simulink library "My_library"  (R2018a)
settings: Solver=VariableStepAuto  StartTime=0.0  StopTime=10.0  RelTol=1e-3  EnableMultiTasking=on
undefined symbols (not defined in the file or in its folder): Ax, Ay, Az, gn, Newton, Nx, Ny, Nz, Raphson, Rx, Ry, Rz, st
libraries: $bdroot x11, simulink x1
(part 2 of 2)

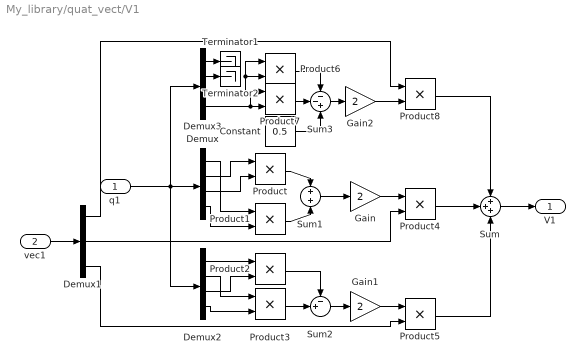
== system My_library/quat_vect/V1 ==
  q1 : Inport
  vec1 : Inport  Port=2
  Constant : Constant  Value=0.5
  Demux : Demux
  Demux1 : Demux  Outputs=3
  Demux2 : Demux
  Demux3 : Demux
  Gain : Gain  Gain=2
  Gain1 : Gain  Gain=2
  Gain2 : Gain  Gain=2
  Product{,1..8} (9 alike) : Product  RndMeth=Zero
  Sum : Sum  Inputs=3
  Sum1 : Sum  Inputs=+|+
  Sum2 : Sum  Inputs=-+|
  Sum3 : Sum  Inputs=--+
  Terminator1 : Terminator
  Terminator2 : Terminator
  V1 : Outport
  wires:
  q1/1 -> Demux2/1, Demux3/1, Demux/1
  Gain1/1 -> Product5/1
  Demux3/4 -> Product7/1, Product7/2
  Product4/1 -> Sum/2
  Product6/1 -> Sum3/1
  Demux/4 -> Product1/2
  Gain2/1 -> Product8/2
  Demux/3 -> Product/2
  Demux1/3 -> Product5/2
  Product8/1 -> Sum/1
  Demux1/2 -> Product4/2
  Demux/2 -> Product/1
  Demux1/1 -> Product8/1
  Sum1/1 -> Gain/1
  Demux2/3 -> Product2/2
  Demux3/3 -> Product6/2, Product6/1
  Constant/1 -> Sum3/3
  Demux3/2 -> Terminator2/1
  Demux3/1 -> Terminator1/1
  Sum3/1 -> Gain2/1
  Product1/1 -> Sum1/2
  Gain/1 -> Product4/1
  Demux2/4 -> Product3/2
  Demux2/1 -> Product2/1
  Product3/1 -> Sum2/2
  Product7/1 -> Sum3/2
  Demux2/2 -> Product3/1
  Product5/1 -> Sum/3
  Product/1 -> Sum1/1
  Demux/1 -> Product1/1
  Sum2/1 -> Gain1/1
  Sum/1 -> V1/1
  Product2/1 -> Sum2/1
  vec1/1 -> Demux1/1

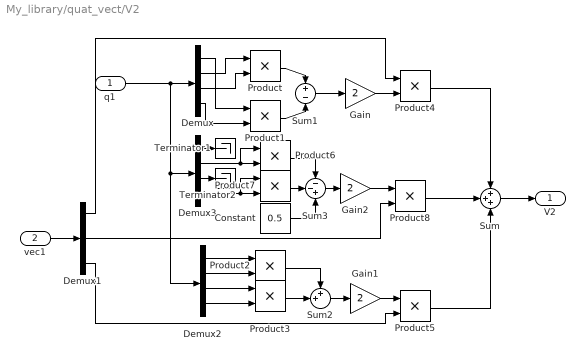
== system My_library/quat_vect/V2 ==
  q1 : Inport
  vec1 : Inport  Port=2
  Constant : Constant  Value=0.5
  Demux : Demux
  Demux1 : Demux  Outputs=3
  Demux2 : Demux
  Demux3 : Demux
  Gain : Gain  Gain=2
  Gain1 : Gain  Gain=2
  Gain2 : Gain  Gain=2
  Product{,1..8} (9 alike) : Product  RndMeth=Zero
  Sum : Sum  Inputs=3
  Sum1 : Sum  Inputs=+|-
  Sum2 : Sum  Inputs=++|
  Sum3 : Sum  Inputs=--+
  Terminator1 : Terminator
  Terminator2 : Terminator
  V2 : Outport
  wires:
  Demux1/2 -> Product8/2
  Product2/1 -> Sum2/1
  Sum3/1 -> Gain2/1
  Demux3/1 -> Terminator1/1
  Demux3/3 -> Terminator2/1
  Product6/1 -> Sum3/1
  Product5/1 -> Sum/3
  vec1/1 -> Demux1/1
  Gain/1 -> Product4/2
  Demux2/4 -> Product3/2
  Product3/1 -> Sum2/2
  Product4/1 -> Sum/1
  Demux/3 -> Product/2
  Demux3/4 -> Product7/2, Product7/1
  Sum/1 -> V2/1
  Demux3/2 -> Product6/1, Product6/2
  Product7/1 -> Sum3/2
  Demux/4 -> Product1/2
  q1/1 -> Demux3/1, Demux2/1, Demux/1
  Gain1/1 -> Product5/1
  Demux1/3 -> Product5/2
  Demux/2 -> Product/1
  Demux2/2 -> Product2/2
  Demux2/3 -> Product3/1
  Gain2/1 -> Product8/1
  Demux1/1 -> Product4/1
  Product/1 -> Sum1/1
  Constant/1 -> Sum3/3
  Product1/1 -> Sum1/2
  Sum1/1 -> Gain/1
  Demux/1 -> Product1/1
  Demux2/1 -> Product2/1
  Product8/1 -> Sum/2
  Sum2/1 -> Gain1/1

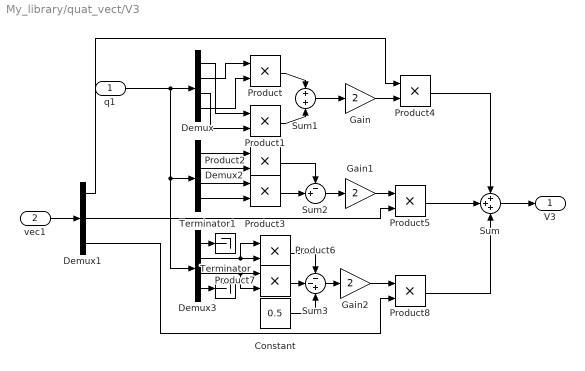
== system My_library/quat_vect/V3 ==
  q1 : Inport
  vec1 : Inport  Port=2
  Constant : Constant  Value=0.5
  Demux : Demux
  Demux1 : Demux  Outputs=3
  Demux2 : Demux
  Demux3 : Demux
  Gain : Gain  Gain=2
  Gain1 : Gain  Gain=2
  Gain2 : Gain  Gain=2
  Product{,1..8} (9 alike) : Product  RndMeth=Zero
  Sum : Sum  Inputs=3
  Sum1 : Sum  Inputs=+|+
  Sum2 : Sum  Inputs=-+|
  Sum3 : Sum  Inputs=--+
  Terminator : Terminator
  Terminator1 : Terminator
  V3 : Outport
  wires:
  Demux3/2 -> Product6/2, Product6/1
  Gain2/1 -> Product8/1
  Sum/1 -> V3/1
  Product1/1 -> Sum1/2
  Sum3/1 -> Gain2/1
  Demux2/1 -> Product2/1
  Product2/1 -> Sum2/1
  Product/1 -> Sum1/1
  Demux/4 -> Product/2
  Demux/2 -> Product/1
  Demux2/2 -> Product2/2
  Demux3/3 -> Product7/1, Product7/2
  Demux2/3 -> Product3/1
  Product8/1 -> Sum/3
  Product3/1 -> Sum2/2
  Product7/1 -> Sum3/2
  Demux2/4 -> Product3/2
  Sum1/1 -> Gain/1
  Demux1/1 -> Product4/1
  q1/1 -> Demux/1, Demux2/1, Demux3/1
  Demux/1 -> Product1/1
  Demux3/4 -> Terminator/1
  Demux/3 -> Product1/2
  Gain/1 -> Product4/2
  Demux1/2 -> Product5/2
  Sum2/1 -> Gain1/1
  Product4/1 -> Sum/1
  Product6/1 -> Sum3/1
  Product5/1 -> Sum/2
  Demux1/3 -> Product8/2
  Demux3/1 -> Terminator1/1
  Gain1/1 -> Product5/1
  Constant/1 -> Sum3/3
  vec1/1 -> Demux1/1

== system My_library/3-axis gyro/Subsystem/No dynamics ==
  In1 : Inport
  Action Port : ActionPort
  Out1 : Outport
  wires:
  In1/1 -> Out1/1

== system My_library/3-axis gyro/Subsystem/Second order dynamics ==
  In1 : Inport
  Action Port : ActionPort
  Demux : Demux  Outputs=3
  Mux : Mux  Inputs=3
  Transfer Fcn X : TransferFcn  Numerator=[w_g*w_g]  Denominator="[1 2*z_g*w_g  w_g*w_g]"
  Transfer Fcn Y : TransferFcn  Numerator=[w_g*w_g]  Denominator="[1 2*z_g*w_g  w_g*w_g]"
  Transfer Fcn Z : TransferFcn  Numerator=[w_g*w_g]  Denominator="[1 2*z_g*w_g  w_g*w_g]"
  Out1 : Outport
  wires:
  Transfer Fcn Z/1 -> Mux/3
  In1/1 -> Demux/1
  Demux/2 -> Transfer Fcn Y/1
  Demux/1 -> Transfer Fcn X/1
  Transfer Fcn Y/1 -> Mux/2
  Transfer Fcn X/1 -> Mux/1
  Demux/3 -> Transfer Fcn Z/1
  Mux/1 -> Out1/1

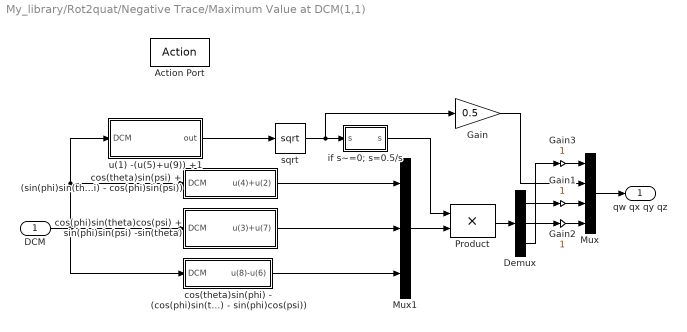
== system My_library/Rot2quat/Negative Trace/Maximum Value at DCM(1,1)  ==
  DCM : Inport
  Action Port : ActionPort
  Demux : Demux  Outputs=3
  Gain : Gain  Gain=0.5  SaturateOnIntegerOverflow=on  OutDataTypeStr=Inherit: Same as input  ParamDataTypeStr=Inherit: Same as input
  Gain1 : Gain  SaturateOnIntegerOverflow=on  OutDataTypeStr=Inherit: Same as input  ParamDataTypeStr=Inherit: Same as input
  Gain2 : Gain  SaturateOnIntegerOverflow=on  OutDataTypeStr=Inherit: Same as input  ParamDataTypeStr=Inherit: Same as input
  Gain3 : Gain  SaturateOnIntegerOverflow=on  OutDataTypeStr=Inherit: Same as input  ParamDataTypeStr=Inherit: Same as input
  Mux : Mux
  Mux1 : Mux  Inputs=3
  Product : Product  SaturateOnIntegerOverflow=on  InputSameDT=on  OutDataTypeStr=Inherit: Same as first input
  cos(phi)sin(theta)cos(psi) + sin(phi)sin(psi) -sin(theta) : Subsystem
  cos(theta)sin(phi) - (cos(phi)sin(theta)sin(psi) - sin(phi)cos(psi)) : Subsystem
  cos(theta)sin(psi) + (sin(phi)sin(theta)cos(psi) - cos(phi)sin(psi)) : Subsystem
  if s~=0; s=0.5/s : Subsystem
  sqrt : Sqrt  AlgorithmType=Newton-Raphson  SaturateOnIntegerOverflow=on
  u(1) -(u(5)+u(9)) +1 : Subsystem
  qw qx qy qz : Outport
  wires:
  DCM/1 -> cos(theta)sin(phi) - (cos(phi)sin(theta)sin(psi) - sin(phi)cos(psi))/1(DCM), cos(phi)sin(theta)cos(psi) + sin(phi)sin(psi) -sin(theta)/1(DCM), cos(theta)sin(psi) + (sin(phi)sin(theta)cos(psi) - cos(phi)sin(psi))/1(DCM), u(1) -(u(5)+u(9)) +1/1(DCM)
  cos(theta)sin(psi) + (sin(phi)sin(theta)cos(psi) - cos(phi)sin(psi))/1(u(4)+u(2)) -> Mux1/1
  cos(phi)sin(theta)cos(psi) + sin(phi)sin(psi) -sin(theta)/1(u(3)+u(7)) -> Mux1/2
  cos(theta)sin(phi) - (cos(phi)sin(theta)sin(psi) - sin(phi)cos(psi))/1(u(8)-u(6)) -> Mux1/3
  Mux/1 -> qw qx qy qz/1
  u(1) -(u(5)+u(9)) +1/1(out) -> sqrt/1
  sqrt/1 -> if s~=0; s=0.5/s/1(s), Gain/1
  Mux1/1 -> Product/2
  Demux/1 -> Gain1/1
  Demux/3 -> Gain3/1
  Demux/2 -> Gain2/1
  Gain1/1 -> Mux/3
  Gain2/1 -> Mux/4
  Gain3/1 -> Mux/1
  Product/1 -> Demux/1
  Gain/1 -> Mux/2
  if s~=0; s=0.5/s/1("s ") -> Product/1

== system My_library/Rot2quat/Negative Trace/Maximum Value at DCM(2,2) ==
  DCM : Inport
  Action Port : ActionPort
  Demux : Demux  Outputs=3
  Gain : Gain  Gain=0.5  SaturateOnIntegerOverflow=on  OutDataTypeStr=Inherit: Same as input  ParamDataTypeStr=Inherit: Same as input
  Gain1 : Gain  SaturateOnIntegerOverflow=on  OutDataTypeStr=Inherit: Same as input  ParamDataTypeStr=Inherit: Same as input
  Gain3 : Gain  SaturateOnIntegerOverflow=on  OutDataTypeStr=Inherit: Same as input  ParamDataTypeStr=Inherit: Same as input
  Gain4 : Gain  SaturateOnIntegerOverflow=on  OutDataTypeStr=Inherit: Same as input  ParamDataTypeStr=Inherit: Same as input
  Mux : Mux
  Mux1 : Mux  Inputs=3
  Product : Product  SaturateOnIntegerOverflow=on  InputSameDT=on  OutDataTypeStr=Inherit: Same as first input
  cos(phi)sin(theta)cos(psi) + sin(phi)sin(psi) +sin(theta) : Subsystem
  cos(theta)sin(phi) + (cos(phi)sin(theta)sin(psi) - sin(phi)cos(psi)) : Subsystem
  cos(theta)sin(psi) + (sin(phi)sin(theta)cos(psi) - cos(phi)sin(psi)) : Subsystem
  if s~=0; s=0.5/s : Subsystem
  sqrt : Sqrt  AlgorithmType=Newton-Raphson  SaturateOnIntegerOverflow=on
  u(5) -(u(1)+u(9)) +1 : Subsystem
  qw qx qy qz : Outport
  wires:
  Mux1/1 -> Product/1
  DCM/1 -> cos(theta)sin(psi) + (sin(phi)sin(theta)cos(psi) - cos(phi)sin(psi))/1(DCM1), cos(theta)sin(phi) + (cos(phi)sin(theta)sin(psi) - sin(phi)cos(psi))/1(DCM1), u(5) -(u(1)+u(9)) +1/1(DCM1), cos(phi)sin(theta)cos(psi) + sin(phi)sin(psi) +sin(theta)/1(DCM1)
  cos(theta)sin(psi) + (sin(phi)sin(theta)cos(psi) - cos(phi)sin(psi))/1(u(4)+u(2)) -> Mux1/1
  cos(theta)sin(phi) + (cos(phi)sin(theta)sin(psi) - sin(phi)cos(psi))/1(u(8)+u(6)) -> Mux1/2
  cos(phi)sin(theta)cos(psi) + sin(phi)sin(psi) +sin(theta)/1(u(3)-u(7)) -> Mux1/3
  Mux/1 -> qw qx qy qz/1
  u(5) -(u(1)+u(9)) +1/1(out) -> sqrt/1
  Gain/1 -> Mux/3
  Product/1 -> Demux/1
  Demux/1 -> Gain1/1
  Demux/2 -> Gain3/1
  Demux/3 -> Gain4/1
  Gain1/1 -> Mux/2
  Gain3/1 -> Mux/4
  Gain4/1 -> Mux/1
  if s~=0; s=0.5/s/1("s ") -> Product/2
  sqrt/1 -> if s~=0; s=0.5/s/1(s), Gain/1

== system My_library/Rot2quat/Negative Trace/Maximum Value at DCM(3,3)  ==
  DCM : Inport
  Action Port : ActionPort
  Demux : Demux  Outputs=3
  Gain : Gain  Gain=0.5  SaturateOnIntegerOverflow=on  OutDataTypeStr=Inherit: Same as input  ParamDataTypeStr=Inherit: Same as input
  Gain1 : Gain  SaturateOnIntegerOverflow=on  OutDataTypeStr=Inherit: Same as input  ParamDataTypeStr=Inherit: Same as input
  Gain2 : Gain  SaturateOnIntegerOverflow=on  OutDataTypeStr=Inherit: Same as input  ParamDataTypeStr=Inherit: Same as input
  Gain3 : Gain  SaturateOnIntegerOverflow=on  OutDataTypeStr=Inherit: Same as input  ParamDataTypeStr=Inherit: Same as input
  Mux : Mux
  Mux1 : Mux  Inputs=3
  Product : Product  SaturateOnIntegerOverflow=on  InputSameDT=on  OutDataTypeStr=Inherit: Same as first input
  cos(phi)sin(theta)cos(psi) + sin(phi)sin(psi) -sin(theta) : Subsystem
  cos(theta)sin(phi) + (cos(phi)sin(theta)sin(psi) - sin(phi)cos(psi)) : Subsystem
  cos(theta)sin(psi) - (sin(phi)sin(theta)cos(psi) - cos(phi)sin(psi)) : Subsystem
  if s~=0; s=0.5/s : Subsystem
  sqrt : Sqrt  AlgorithmType=Newton-Raphson  SaturateOnIntegerOverflow=on
  u(9) -(u(1)+u(5)) +1 : Subsystem
  qw qx qy qz : Outport
  wires:
  Mux1/1 -> Product/1
  DCM/1 -> cos(theta)sin(phi) + (cos(phi)sin(theta)sin(psi) - sin(phi)cos(psi))/1(DCM1), cos(phi)sin(theta)cos(psi) + sin(phi)sin(psi) -sin(theta)/1(DCM1), u(9) -(u(1)+u(5)) +1/1(DCM1), cos(theta)sin(psi) - (sin(phi)sin(theta)cos(psi) - cos(phi)sin(psi))/1(DCM1)
  cos(phi)sin(theta)cos(psi) + sin(phi)sin(psi) -sin(theta)/1(u(3)+u(7)) -> Mux1/1
  cos(theta)sin(phi) + (cos(phi)sin(theta)sin(psi) - sin(phi)cos(psi))/1(u(8)+u(6)) -> Mux1/2
  cos(theta)sin(psi) - (sin(phi)sin(theta)cos(psi) - cos(phi)sin(psi))/1(u(4)-u(2)) -> Mux1/3
  Mux/1 -> qw qx qy qz/1
  u(9) -(u(1)+u(5)) +1/1(out) -> sqrt/1
  sqrt/1 -> if s~=0; s=0.5/s/1(s), Gain/1
  Product/1 -> Demux/1
  Demux/1 -> Gain1/1
  Demux/3 -> Gain3/1
  Demux/2 -> Gain2/1
  Gain/1 -> Mux/4
  Gain1/1 -> Mux/2
  Gain2/1 -> Mux/3
  Gain3/1 -> Mux/1
  if s~=0; s=0.5/s/1("s ") -> Product/2

== system My_library/Rot2quat/Negative Trace/diag(DCM) ==
  DCM : Inport
  Demux : Demux  Outputs=3
  Selector : Selector  InputPortWidth=9  IndexOptions=Index vector (dialog)  Indices=[1 5 9]  OutputSizes=1
  u(1) : Outport
  u(5) : Outport  Port=2
  u(9) : Outport  Port=3
  wires:
  DCM/1 -> Selector/1
  Demux/3 -> u(9)/1
  Selector/1 -> Demux/1
  Demux/1 -> u(1)/1
  Demux/2 -> u(5)/1

== system My_library/Rot2quat/Positive Trace/cos(phi)sin(theta)cos(psi) + sin(phi)sin(psi) +sin(theta) ==
  DCM : Inport
  Add1 : Sum  Inputs=+-|
  Demux1 : Demux  Outputs=2
  Selector1 : Selector  InputPortWidth=9  IndexOptions=Index vector (dialog)  Indices=[3 7]  OutputSizes=1
  u(3)-u(7) : Outport
  wires:
  DCM/1 -> Selector1/1
  Demux1/1 -> Add1/1
  Demux1/2 -> Add1/2
  Selector1/1 -> Demux1/1
  Add1/1 -> u(3)-u(7)/1

== system My_library/Rot2quat/Positive Trace/cos(theta)sin(phi) - (cos(phi)sin(theta)sin(psi) - sin(phi)cos(psi))1 ==
  DCM : Inport
  Add : Sum  Inputs=|-+
  Demux : Demux  Outputs=2
  Selector : Selector  InputPortWidth=9  IndexOptions=Index vector (dialog)  Indices=[6 8]  OutputSizes=1
  u(8)-u(6) : Outport
  wires:
  DCM/1 -> Selector/1
  Add/1 -> u(8)-u(6)/1
  Selector/1 -> Demux/1
  Demux/2 -> Add/2
  Demux/1 -> Add/1

== system My_library/Rot2quat/Positive Trace/cos(theta)sin(psi) - (sin(phi)sin(theta)cos(psi) - cos(phi)sin(psi))1 ==
  DCM : Inport
  Add2 : Sum  Inputs=|-+
  Demux2 : Demux  Outputs=2
  Selector2 : Selector  InputPortWidth=9  IndexOptions=Index vector (dialog)  Indices=[2 4]  OutputSizes=1
  u(4)-u(2) : Outport
  wires:
  Add2/1 -> u(4)-u(2)/1
  Selector2/1 -> Demux2/1
  DCM/1 -> Selector2/1
  Demux2/2 -> Add2/2
  Demux2/1 -> Add2/1

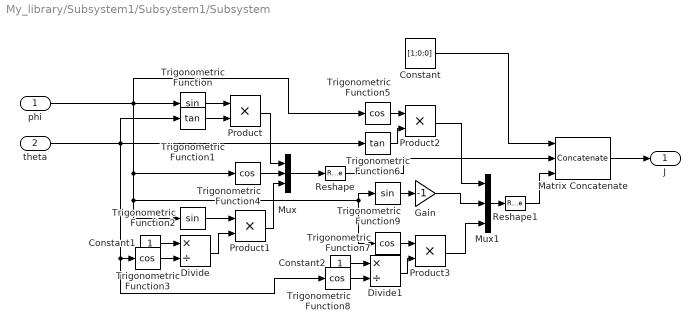
== system My_library/Subsystem1/Subsystem1/Subsystem ==
  phi : Inport
  theta : Inport  Port=2
  Constant : Constant  Value=[1;0;0]
  Constant1 : Constant
  Constant2 : Constant
  Divide : Product  Inputs=*/
  Divide1 : Product  Inputs=*/
  Gain : Gain  Gain=-1
  Matrix Concatenate : Concatenate  NumInputs=3  Mode=Multidimensional array  ConcatenateDimension=2
  Mux : Mux  Inputs=3
  Mux1 : Mux  Inputs=3
  Product{,1..3} (4 alike) : Product
  Reshape : Reshape
  Reshape1 : Reshape
  Trigonometric Function : Trigonometry
  Trigonometric Function1 : Trigonometry  Operator=tan
  Trigonometric Function2 : Trigonometry
  Trigonometric Function{3..5,7..8} (5 alike) : Trigonometry  Operator=cos
  Trigonometric Function6 : Trigonometry  Operator=tan
  Trigonometric Function9 : Trigonometry
  J : Outport
  wires:
  Reshape1/1 -> Matrix Concatenate/3
  Reshape/1 -> Matrix Concatenate/2
  Mux1/1 -> Reshape1/1
  Product3/1 -> Mux1/3
  Mux/1 -> Reshape/1
  theta/1 -> Trigonometric Function6/1, Trigonometric Function1/1, Trigonometric Function8/1, Trigonometric Function3/1
  Gain/1 -> Mux1/2
  Constant1/1 -> Divide/1
  Divide/1 -> Product1/2
  Trigonometric Function1/1 -> Product/2
  phi/1 -> Trigonometric Function7/1, Trigonometric Function9/1, Trigonometric Function2/1, Trigonometric Function4/1, Trigonometric Function/1, Trigonometric Function5/1
  Trigonometric Function9/1 -> Gain/1
  Trigonometric Function7/1 -> Product3/1
  Divide1/1 -> Product3/2
  Trigonometric Function6/1 -> Product2/2
  Trigonometric Function5/1 -> Product2/1
  Product/1 -> Mux/1
  Trigonometric Function/1 -> Product/1
  Trigonometric Function8/1 -> Divide1/2
  Constant2/1 -> Divide1/1
  Product1/1 -> Mux/3
  Matrix Concatenate/1 -> J/1
  Trigonometric Function4/1 -> Mux/2
  Constant/1 -> Matrix Concatenate/1
  Trigonometric Function2/1 -> Product1/1
  Product2/1 -> Mux1/1
  Trigonometric Function3/1 -> Divide/2

== system My_library/quat_normalise/quat_modulus /q_norm ==
  q : Inport
  Demux : Demux
  Product{1..4} (4 alike) : Product
  Sum : Sum  Inputs=4
  norm(q) : Outport
  wires:
  Demux/1 -> Product1/1, Product1/2
  Demux/3 -> Product3/1, Product3/2
  Demux/2 -> Product2/1, Product2/2
  Product3/1 -> Sum/3
  Product4/1 -> Sum/4
  Product1/1 -> Sum/1
  Demux/4 -> Product4/1, Product4/2
  Product2/1 -> Sum/2
  q/1 -> Demux/1
  Sum/1 -> norm(q)/1

== system My_library/Rot2quat/Negative Trace/Maximum Value at DCM(1,1) /cos(phi)sin(theta)cos(psi) + sin(phi)sin(psi) -sin(theta) ==
  DCM : Inport
  Add : Sum  Inputs=++|
  Demux1 : Demux  Outputs=2
  Selector : Selector  InputPortWidth=9  IndexOptions=Index vector (dialog)  Indices=[3 7]  OutputSizes=1
  u(3)+u(7) : Outport
  wires:
  Demux1/2 -> Add/2
  DCM/1 -> Selector/1
  Selector/1 -> Demux1/1
  Demux1/1 -> Add/1
  Add/1 -> u(3)+u(7)/1

== system My_library/Rot2quat/Negative Trace/Maximum Value at DCM(1,1) /cos(theta)sin(phi) - (cos(phi)sin(theta)sin(psi) - sin(phi)cos(psi)) ==
  DCM : Inport
  Add : Sum  Inputs=|-+
  Demux1 : Demux  Outputs=2
  Selector : Selector  InputPortWidth=9  IndexOptions=Index vector (dialog)  Indices=[6 8]  OutputSizes=1
  u(8)-u(6) : Outport
  wires:
  DCM/1 -> Selector/1
  Selector/1 -> Demux1/1
  Add/1 -> u(8)-u(6)/1
  Demux1/2 -> Add/2
  Demux1/1 -> Add/1

== system My_library/Rot2quat/Negative Trace/Maximum Value at DCM(1,1) /cos(theta)sin(psi) + (sin(phi)sin(theta)cos(psi) - cos(phi)sin(psi)) ==
  DCM : Inport
  Add : Sum  Inputs=|++
  Demux1 : Demux  Outputs=2
  Selector : Selector  InputPortWidth=9  IndexOptions=Index vector (dialog)  Indices=[2 4]  OutputSizes=1
  u(4)+u(2) : Outport
  wires:
  Demux1/1 -> Add/1
  DCM/1 -> Selector/1
  Selector/1 -> Demux1/1
  Add/1 -> u(4)+u(2)/1
  Demux1/2 -> Add/2

== system My_library/Rot2quat/Negative Trace/Maximum Value at DCM(1,1) /if s~=0; s=0.5//s ==
  s : Inport
  Constant1 : Constant  Value=0.5  OutDataTypeStr=Inherit: Inherit via back propagation
  Constant2 : Constant  Value=[0 1]  OutDataTypeStr=Inherit: Inherit via back propagation
  Demux1 : Demux  Outputs=2
  Mux2 : Mux  Inputs=2
  Product1 : Product  Inputs=*/  RndMeth=Zero
  Switch : Switch  Criteria=u2 ~= 0  SaturateOnIntegerOverflow=on  InputSameDT=on
  "s " : Outport
  wires:
  Demux1/2 -> Product1/2
  Switch/1 -> Demux1/1
  Constant2/1 -> Switch/3
  Product1/1 -> "s "/1
  s/1 -> Switch/2, Mux2/2
  Demux1/1 -> Product1/1
  Constant1/1 -> Mux2/1
  Mux2/1 -> Switch/1

== system My_library/Rot2quat/Negative Trace/Maximum Value at DCM(1,1) /u(1) -(u(5)+u(9)) +1 ==
  DCM : Inport
  Add : Sum  Inputs=+--+
  Constant : Constant  OutDataTypeStr=Inherit: Inherit via back propagation
  Demux1 : Demux  Outputs=3
  Selector : Selector  InputPortWidth=9  IndexOptions=Index vector (dialog)  Indices=[1 5 9]  OutputSizes=1
  out : Outport
  wires:
  Add/1 -> out/1
  Constant/1 -> Add/4
  Selector/1 -> Demux1/1
  Demux1/1 -> Add/1
  Demux1/2 -> Add/2
  DCM/1 -> Selector/1
  Demux1/3 -> Add/3

== system My_library/Rot2quat/Negative Trace/Maximum Value at DCM(2,2)/cos(phi)sin(theta)cos(psi) + sin(phi)sin(psi) +sin(theta) ==
  DCM1 : Inport
  Add : Sum  Inputs=+-|
  Demux1 : Demux  Outputs=2
  Selector : Selector  InputPortWidth=9  IndexOptions=Index vector (dialog)  Indices=[3 7]  OutputSizes=1
  u(3)-u(7) : Outport
  wires:
  DCM1/1 -> Selector/1
  Selector/1 -> Demux1/1
  Add/1 -> u(3)-u(7)/1
  Demux1/1 -> Add/1
  Demux1/2 -> Add/2

== system My_library/Rot2quat/Negative Trace/Maximum Value at DCM(2,2)/cos(theta)sin(phi) + (cos(phi)sin(theta)sin(psi) - sin(phi)cos(psi)) ==
  DCM1 : Inport
  Add : Sum  Inputs=|++
  Demux1 : Demux  Outputs=2
  Selector : Selector  InputPortWidth=9  IndexOptions=Index vector (dialog)  Indices=[6 8]  OutputSizes=1
  u(8)+u(6) : Outport
  wires:
  DCM1/1 -> Selector/1
  Selector/1 -> Demux1/1
  Demux1/2 -> Add/2
  Add/1 -> u(8)+u(6)/1
  Demux1/1 -> Add/1

== system My_library/Rot2quat/Negative Trace/Maximum Value at DCM(2,2)/cos(theta)sin(psi) + (sin(phi)sin(theta)cos(psi) - cos(phi)sin(psi)) ==
  DCM1 : Inport
  Add : Sum  Inputs=|++
  Demux1 : Demux  Outputs=2
  Selector : Selector  InputPortWidth=9  IndexOptions=Index vector (dialog)  Indices=[2 4]  OutputSizes=1
  u(4)+u(2) : Outport
  wires:
  Demux1/1 -> Add/1
  Add/1 -> u(4)+u(2)/1
  DCM1/1 -> Selector/1
  Selector/1 -> Demux1/1
  Demux1/2 -> Add/2

== system My_library/Rot2quat/Negative Trace/Maximum Value at DCM(2,2)/if s~=0; s=0.5//s ==
  s : Inport
  Constant1 : Constant  Value=0.5  OutDataTypeStr=Inherit: Inherit via back propagation
  Constant2 : Constant  Value=[0 1]  OutDataTypeStr=Inherit: Inherit via back propagation
  Demux1 : Demux  Outputs=2
  Mux2 : Mux  Inputs=2
  Product1 : Product  Inputs=*/  RndMeth=Zero
  Switch : Switch  Criteria=u2 ~= 0  SaturateOnIntegerOverflow=on  InputSameDT=on
  "s " : Outport
  wires:
  Demux1/2 -> Product1/2
  Mux2/1 -> Switch/1
  Switch/1 -> Demux1/1
  Constant1/1 -> Mux2/1
  s/1 -> Switch/2, Mux2/2
  Product1/1 -> "s "/1
  Constant2/1 -> Switch/3
  Demux1/1 -> Product1/1

== system My_library/Rot2quat/Negative Trace/Maximum Value at DCM(2,2)/u(5) -(u(1)+u(9)) +1 ==
  DCM1 : Inport
  Add : Sum  Inputs=-+-+
  Constant : Constant  OutDataTypeStr=Inherit: Inherit via back propagation
  Demux1 : Demux  Outputs=3
  Selector : Selector  InputPortWidth=9  IndexOptions=Index vector (dialog)  Indices=[1 5 9]  OutputSizes=1
  out : Outport
  wires:
  DCM1/1 -> Selector/1
  Demux1/1 -> Add/1
  Selector/1 -> Demux1/1
  Demux1/2 -> Add/2
  Add/1 -> out/1
  Constant/1 -> Add/4
  Demux1/3 -> Add/3

== system My_library/Rot2quat/Negative Trace/Maximum Value at DCM(3,3) /cos(phi)sin(theta)cos(psi) + sin(phi)sin(psi) -sin(theta) ==
  DCM1 : Inport
  Add : Sum  Inputs=++|
  Demux1 : Demux  Outputs=2
  Selector : Selector  InputPortWidth=9  IndexOptions=Index vector (dialog)  Indices=[3 7]  OutputSizes=1
  u(3)+u(7) : Outport
  wires:
  Demux1/2 -> Add/2
  Demux1/1 -> Add/1
  DCM1/1 -> Selector/1
  Add/1 -> u(3)+u(7)/1
  Selector/1 -> Demux1/1

== system My_library/Rot2quat/Negative Trace/Maximum Value at DCM(3,3) /cos(theta)sin(phi) + (cos(phi)sin(theta)sin(psi) - sin(phi)cos(psi)) ==
  DCM1 : Inport
  Add : Sum  Inputs=|++
  Demux1 : Demux  Outputs=2
  Selector : Selector  InputPortWidth=9  IndexOptions=Index vector (dialog)  Indices=[6 8]  OutputSizes=1
  u(8)+u(6) : Outport
  wires:
  Add/1 -> u(8)+u(6)/1
  Demux1/1 -> Add/1
  DCM1/1 -> Selector/1
  Selector/1 -> Demux1/1
  Demux1/2 -> Add/2

== system My_library/Rot2quat/Negative Trace/Maximum Value at DCM(3,3) /cos(theta)sin(psi) - (sin(phi)sin(theta)cos(psi) - cos(phi)sin(psi)) ==
  DCM1 : Inport
  Add : Sum  Inputs=|-+
  Demux1 : Demux  Outputs=2
  Selector : Selector  InputPortWidth=9  IndexOptions=Index vector (dialog)  Indices=[2 4]  OutputSizes=1
  u(4)-u(2) : Outport
  wires:
  Add/1 -> u(4)-u(2)/1
  Demux1/2 -> Add/2
  Selector/1 -> Demux1/1
  Demux1/1 -> Add/1
  DCM1/1 -> Selector/1

== system My_library/Rot2quat/Negative Trace/Maximum Value at DCM(3,3) /if s~=0; s=0.5//s ==
  s : Inport
  Constant1 : Constant  Value=0.5  OutDataTypeStr=Inherit: Inherit via back propagation
  Constant2 : Constant  Value=[0 1]  OutDataTypeStr=Inherit: Inherit via back propagation
  Demux1 : Demux  Outputs=2
  Mux2 : Mux  Inputs=2
  Product1 : Product  Inputs=*/  RndMeth=Zero
  Switch : Switch  Criteria=u2 ~= 0  SaturateOnIntegerOverflow=on  InputSameDT=on
  "s " : Outport
  wires:
  Mux2/1 -> Switch/1
  Demux1/2 -> Product1/2
  Constant1/1 -> Mux2/1
  Product1/1 -> "s "/1
  Demux1/1 -> Product1/1
  Constant2/1 -> Switch/3
  s/1 -> Mux2/2, Switch/2
  Switch/1 -> Demux1/1

== system My_library/Rot2quat/Negative Trace/Maximum Value at DCM(3,3) /u(9) -(u(1)+u(5)) +1 ==
  DCM1 : Inport
  Add : Sum  Inputs=--++
  Constant : Constant  OutDataTypeStr=Inherit: Inherit via back propagation
  Demux1 : Demux  Outputs=3
  Selector : Selector  InputPortWidth=9  IndexOptions=Index vector (dialog)  Indices=[1 5 9]  OutputSizes=1
  out : Outport
  wires:
  Demux1/3 -> Add/3
  Demux1/1 -> Add/1
  Selector/1 -> Demux1/1
  Demux1/2 -> Add/2
  DCM1/1 -> Selector/1
  Add/1 -> out/1
  Constant/1 -> Add/4

== matlab function My_library/Control_Switch /MATLAB Function2 ==
  data: x input; yes output
function yes = control_switch(x)
%#codegen

yes=0;
w = x(5:7);

if w(1)>=-0.0087 && w(1)<=0.0087 
    t1=0;
else
    t1=1;
end

if w(2)>=-0.0087 && w(2)<=0.0087 
    t2=0;
else
    t2=1;
end

if w(3)>=-0.0087 && w(3)<=0.0087 
    t3=0;
else
    t3=1;
end

if (t1+t2+t3==0)
    yes = 1;
else
    yes=0;
end
